simulink model "parallel_modules_2_parasitic"  (R2018a)
settings: Solver=FixedStepDiscrete  StartTime=0.0  StopTime=Tfinal  FixedStep=SampleTime  RelTol=1e-3
values from neighbouring files (symbols this model uses):
  C1A = 5e-6    (= 5e-06)    [param_parallel_modules_2_parasitic.m]
  C1B = 5e-6    (= 5e-06)    [param_parallel_modules_2_parasitic.m]
  C1C = 5e-6    (= 5e-06)    [param_parallel_modules_2_parasitic.m]
  connector_ind = 0.6e-6    (= 6e-07)    [param_parallel_modules_2_parasitic.m]
  connector_ind1 = 0.6e-6    (= 6e-07)    [param_parallel_modules_2_parasitic.m]
  connector_ind2 = 1.2e-6    (= 1.2e-06)    [param_parallel_modules_2_parasitic.m]
  connector_res = 1e-3    (= 0.001)    [param_parallel_modules_2_parasitic.m]
  connector_res1 = 1e-3    (= 0.001)    [param_parallel_modules_2_parasitic.m]
  connector_res2 = 1e-3    (= 0.001)    [param_parallel_modules_2_parasitic.m]
  ESLA = 19e-9    (= 1.9e-08)    [param_parallel_modules_2_parasitic.m]
  ESLB = 19e-9    (= 1.9e-08)    [param_parallel_modules_2_parasitic.m]
  ESLC = 19e-9    (= 1.9e-08)    [param_parallel_modules_2_parasitic.m]
  ESRA = 21.1e-3    (= 0.0211)    [param_parallel_modules_2_parasitic.m]
  ESRB = 21.1e-3    (= 0.0211)    [param_parallel_modules_2_parasitic.m]
  ESRC = 21.1e-3    (= 0.0211)    [param_parallel_modules_2_parasitic.m]
  ffund = 50    [param_parallel_modules_2_parasitic.m]
  LABBot = 10.20e-9    (= 1.02e-08)    [param_parallel_modules_2_parasitic.m]
  LABot = 20.25e-9    (= 2.025e-08)    [param_parallel_modules_2_parasitic.m]
  LABTop = 18.30e-9    (= 1.83e-08)    [param_parallel_modules_2_parasitic.m]
  LAMid = 01.30e-9    (= 1.3e-09)    [param_parallel_modules_2_parasitic.m]
  LATop = 03.40e-9    (= 3.4e-09)    [param_parallel_modules_2_parasitic.m]
  LBBot = 20.38e-9    (= 2.038e-08)    [param_parallel_modules_2_parasitic.m]
  LBCBot = 11.14e-9    (= 1.114e-08)    [param_parallel_modules_2_parasitic.m]
  LBCTop = 21.84e-9    (= 2.184e-08)    [param_parallel_modules_2_parasitic.m]
  LBMid = 01.30e-9    (= 1.3e-09)    [param_parallel_modules_2_parasitic.m]
  LBTop = 03.38e-9    (= 3.38e-09)    [param_parallel_modules_2_parasitic.m]
  LCBot = 20.94e-9    (= 2.094e-08)    [param_parallel_modules_2_parasitic.m]
  LCMid = 01.30e-9    (= 1.3e-09)    [param_parallel_modules_2_parasitic.m]
  LCTop = 03.41e-9    (= 3.41e-09)    [param_parallel_modules_2_parasitic.m]
  Lin = 1e-6    (= 1e-06)    [param_parallel_modules_2_parasitic.m]
  Lload1 = Xload1/(2*pi*ffund)    [param_parallel_modules_2_parasitic.m]
  Lload2 = Xload2/(2*pi*ffund)    [param_parallel_modules_2_parasitic.m]
  ModulationIndex1 = 0.9    [param_parallel_modules_2_parasitic.m]
  ModulationIndex2 = 0.9    [param_parallel_modules_2_parasitic.m]
  Module1Phase = 0    [param_parallel_modules_2_parasitic.m]
  Module2Phase = 0    [param_parallel_modules_2_parasitic.m]
  RABBot = 1422e-6-662e-6    (= 0.00076)    [param_parallel_modules_2_parasitic.m]
  RABot = 6645e-6    (= 0.006645)    [param_parallel_modules_2_parasitic.m]
  RABTop = 1037e-6-611e-6    (= 0.000426)    [param_parallel_modules_2_parasitic.m]
  RAMid = 218.8e-6*2    (= 0.0004376)    [param_parallel_modules_2_parasitic.m]
  RATop = 854e-6    (= 0.000854)    [param_parallel_modules_2_parasitic.m]
  RBBot = 664e-6    (= 0.000664)    [param_parallel_modules_2_parasitic.m]
  RBCBot = 662e-6-595e-6    (= 6.7e-05)    [param_parallel_modules_2_parasitic.m]
  RBCTop = 867e-6-611e-6    (= 0.000256)    [param_parallel_modules_2_parasitic.m]
  RBMid = 218e-6*2    (= 0.000436)    [param_parallel_modules_2_parasitic.m]
  RBTop = 813e-6    (= 0.000813)    [param_parallel_modules_2_parasitic.m]
  RCBot = 664e-6    (= 0.000664)    [param_parallel_modules_2_parasitic.m]
  RCMid = 218.3e-6*2    (= 0.0004366)    [param_parallel_modules_2_parasitic.m]
  RCTop = 854e-6    (= 0.000854)    [param_parallel_modules_2_parasitic.m]
  Rin = 0.1    [param_parallel_modules_2_parasitic.m]
  Rload1 = Z1*PF1    [param_parallel_modules_2_parasitic.m]
  Rload2 = Z2*PF2    [param_parallel_modules_2_parasitic.m]
  SampleTime = 1e-8    (= 1e-08)    [param_parallel_modules_2_parasitic.m]
  Vin = Vdc + Idc*Rin+((Idc1*connector_res1+Idc2*connector_res2)/2)    (= 271.488888889)    [param_parallel_modules_2_parasitic.m]
libraries: powerlib x90, simulink x12, powerlib_meascontrol x2
settings Model: Creator=enes_  LastModifiedBy=enes_

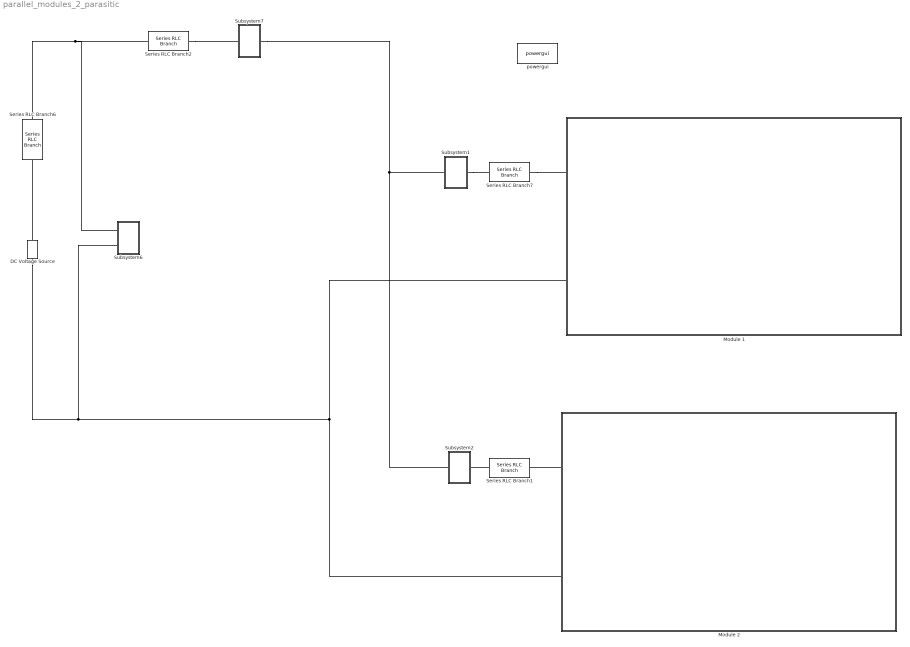
== system parallel_modules_2_parasitic ==
  DC Voltage Source : powerlib/Electrical Sources/DC Voltage Source  Amplitude=Vin  Measurements=None
  Module 1 : Subsystem
  Module 2 : Subsystem
  Series RLC Branch1 : powerlib/Elements/Series RLC Branch  LConnTagsString=__new0  RConnTagsString=__new0  BranchType=RL  Resistance=connector_res2  Inductance=connector_ind2  SetiL0=off  InitialCurrent=0  Capacitance=1e-6  Setx0=off  InitialVoltage=0  Measurements=None
  Series RLC Branch2 : powerlib/Elements/Series RLC Branch  LConnTagsString=__new0  RConnTagsString=__new0  BranchType=RL  Resistance=connector_res  Inductance=connector_ind  SetiL0=off  InitialCurrent=0  Capacitance=1e-6  Setx0=off  InitialVoltage=0  Measurements=None
  Series RLC Branch6 : powerlib/Elements/Series RLC Branch  LConnTagsString=__new0  RConnTagsString=__new0  BranchType=RL  Resistance=Rin  Inductance=Lin  SetiL0=off  InitialCurrent=0  Capacitance=C1A  Setx0=off  InitialVoltage=0  Measurements=None
  Series RLC Branch7 : powerlib/Elements/Series RLC Branch  LConnTagsString=__new0  RConnTagsString=__new0  BranchType=RL  Resistance=connector_res1  Inductance=connector_ind1  SetiL0=off  InitialCurrent=0  Capacitance=1e-6  Setx0=off  InitialVoltage=0  Measurements=None
  Subsystem1 : Subsystem
  Subsystem2 : Subsystem
  Subsystem6 : Subsystem
  Subsystem7 : Subsystem
  powergui : powerlib/powergui  Priority=1  SimulationMode=Discrete  SampleTime=SampleTime  frequency=60  Iterations=50  frequencyindice=0  Pbase=100e6  ErrMax=1e-4  UnitsV=kV  UnitsW=MW  buscounter=0  FunctionMessages=off  echomessages=off  EnableUseOfTLC=off  CurrentSourceSwitches=off  DisableSnubberDevices=off  DisableRonSwitches=off  DisableVfSwitches=off  DisplayEquations=off  SolverType=Tustin/Backward Euler (TBE)  Interpol=off  ExternalGateDelay=off  methode=off  Ts=100  x0status=blocks  SPID=off  SwTol=0  HookPort=off  RestoreLinks=warning  ResistiveCurrentMeasurement=off  Frange=[0:2:500]  Ylog=off  Xlog=on  ShowGrid=off  save=off  variable=ZData  structure=0  ZoomFFT=off  StartTime=0.0  cycles=1  DisplayStyle=1  fundamental=60  FreqAxis=off  MaxFrequency=1000  frequencyindicesteady=1  RmsSteady=1  display=off
  connections:
  DC Voltage Source/RConn1 -- Series RLC Branch6/RConn1
  Subsystem6/LConn1 -- Series RLC Branch2/LConn1 -- Series RLC Branch6/LConn1
  Subsystem6/LConn2 -- DC Voltage Source/LConn1 -- Module 1/LConn2 -- Module 2/LConn2
  Subsystem7/LConn1 -- Subsystem2/RConn1 -- Subsystem1/RConn1
  Series RLC Branch7/RConn1 -- Module 1/LConn1
  Module 2/LConn1 -- Series RLC Branch1/RConn1
  Series RLC Branch2/RConn1 -- Subsystem7/RConn1
  Subsystem1/LConn1 -- Series RLC Branch7/LConn1
  Series RLC Branch1/LConn1 -- Subsystem2/LConn1

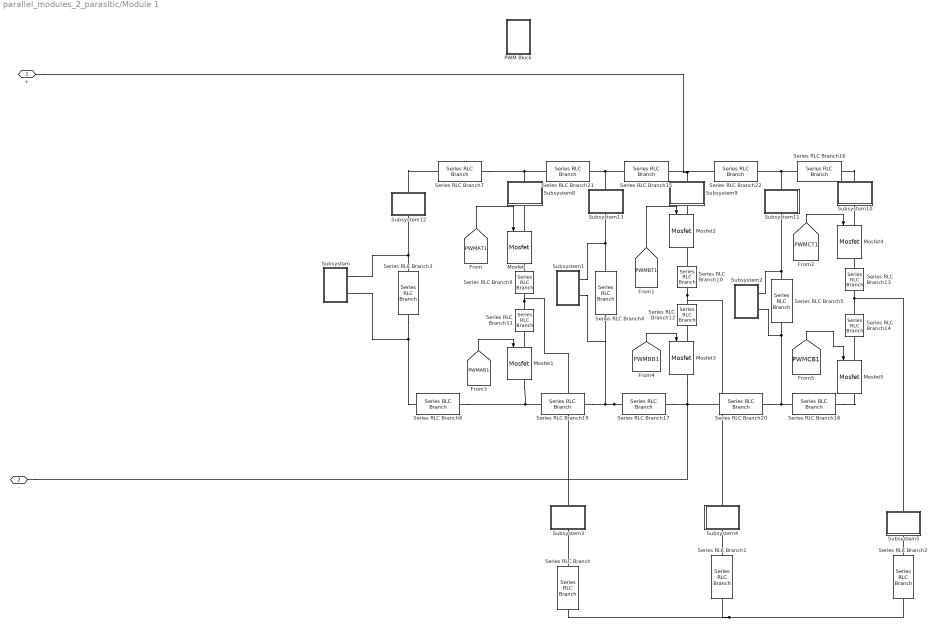
== system parallel_modules_2_parasitic/Module 1 ==
  Mosfet{,1..5} (6 alike) : powerlib/Power Electronics/Mosfet  Ron=0.1  Lon=0  Rd=0.01  Vfd=0  IC=0  Rs=1e5  Cs=inf  Measurements=on
  PWM Block : Subsystem
  Series RLC Branch : powerlib/Elements/Series RLC Branch  LConnTagsString=__new0  RConnTagsString=__new0  BranchType=RL  Resistance=Rload1  Inductance=Lload1  SetiL0=off  InitialCurrent=0  Capacitance=1e-6  Setx0=off  InitialVoltage=0  Measurements=None
  Series RLC Branch1 : powerlib/Elements/Series RLC Branch  LConnTagsString=__new0  RConnTagsString=__new0  BranchType=RL  Resistance=Rload1  Inductance=Lload1  SetiL0=off  InitialCurrent=0  Capacitance=1e-6  Setx0=off  InitialVoltage=0  Measurements=None
  Series RLC Branch10 : powerlib/Elements/Series RLC Branch  LConnTagsString=__new0  RConnTagsString=__new0  BranchType=RL  Resistance=RBMid/2  Inductance=LBMid/2  SetiL0=off  InitialCurrent=0  Capacitance=1e-6  Setx0=off  InitialVoltage=0  Measurements=None
  Series RLC Branch11 : powerlib/Elements/Series RLC Branch  LConnTagsString=__new0  RConnTagsString=__new0  BranchType=RL  Resistance=RAMid/2  Inductance=LAMid/2  SetiL0=off  InitialCurrent=0  Capacitance=1e-6  Setx0=off  InitialVoltage=0  Measurements=None
  Series RLC Branch12 : powerlib/Elements/Series RLC Branch  LConnTagsString=__new0  RConnTagsString=__new0  BranchType=RL  Resistance=RBMid/2  Inductance=LBMid/2  SetiL0=off  InitialCurrent=0  Capacitance=1e-6  Setx0=off  InitialVoltage=0  Measurements=None
  Series RLC Branch13 : powerlib/Elements/Series RLC Branch  LConnTagsString=__new0  RConnTagsString=__new0  BranchType=RL  Resistance=RCMid/2  Inductance=LCMid/2  SetiL0=off  InitialCurrent=0  Capacitance=1e-6  Setx0=off  InitialVoltage=0  Measurements=None
  Series RLC Branch14 : powerlib/Elements/Series RLC Branch  LConnTagsString=__new0  RConnTagsString=__new0  BranchType=RL  Resistance=RCMid/2  Inductance=LCMid/2  SetiL0=off  InitialCurrent=0  Capacitance=1e-6  Setx0=off  InitialVoltage=0  Measurements=None
  Series RLC Branch15 : powerlib/Elements/Series RLC Branch  LConnTagsString=__new0  RConnTagsString=__new0  BranchType=RL  Resistance=RBTop  Inductance=LBTop  SetiL0=off  InitialCurrent=0  Capacitance=1e-6  Setx0=off  InitialVoltage=0  Measurements=None
  Series RLC Branch16 : powerlib/Elements/Series RLC Branch  LConnTagsString=__new0  RConnTagsString=__new0  BranchType=RL  Resistance=RCTop  Inductance=LCTop  SetiL0=off  InitialCurrent=0  Capacitance=1e-6  Setx0=off  InitialVoltage=0  Measurements=None
  Series RLC Branch17 : powerlib/Elements/Series RLC Branch  LConnTagsString=__new0  RConnTagsString=__new0  BranchType=RL  Resistance=RBBot  Inductance=LBBot  SetiL0=off  InitialCurrent=0  Capacitance=1e-6  Setx0=off  InitialVoltage=0  Measurements=None
  Series RLC Branch18 : powerlib/Elements/Series RLC Branch  LConnTagsString=__new0  RConnTagsString=__new0  BranchType=RL  Resistance=RCBot  Inductance=LCBot  SetiL0=off  InitialCurrent=0  Capacitance=1e-6  Setx0=off  InitialVoltage=0  Measurements=None
  Series RLC Branch19 : powerlib/Elements/Series RLC Branch  LConnTagsString=__new0  RConnTagsString=__new0  BranchType=RL  Resistance=RABBot  Inductance=LABBot  SetiL0=off  InitialCurrent=0  Capacitance=1e-6  Setx0=off  InitialVoltage=0  Measurements=None
  Series RLC Branch2 : powerlib/Elements/Series RLC Branch  LConnTagsString=__new0  RConnTagsString=__new0  BranchType=RL  Resistance=Rload1  Inductance=Lload1  SetiL0=off  InitialCurrent=0  Capacitance=1e-6  Setx0=off  InitialVoltage=0  Measurements=None
  Series RLC Branch20 : powerlib/Elements/Series RLC Branch  LConnTagsString=__new0  RConnTagsString=__new0  BranchType=RL  Resistance=RBCBot  Inductance=LBCBot  SetiL0=off  InitialCurrent=0  Capacitance=1e-6  Setx0=off  InitialVoltage=0  Measurements=None
  Series RLC Branch21 : powerlib/Elements/Series RLC Branch  LConnTagsString=__new0  RConnTagsString=__new0  BranchType=RL  Resistance=RABTop  Inductance=LABTop  SetiL0=off  InitialCurrent=0  Capacitance=1e-6  Setx0=off  InitialVoltage=0  Measurements=None
  Series RLC Branch22 : powerlib/Elements/Series RLC Branch  LConnTagsString=__new0  RConnTagsString=__new0  BranchType=RL  Resistance=RBCTop  Inductance=LBCTop  SetiL0=off  InitialCurrent=0  Capacitance=1e-6  Setx0=off  InitialVoltage=0  Measurements=None
  Series RLC Branch3 : powerlib/Elements/Series RLC Branch  LConnTagsString=__new0  RConnTagsString=__new0  BranchType=RLC  Resistance=ESRA  Inductance=ESLA  SetiL0=off  InitialCurrent=0  Capacitance=C1A  Setx0=off  InitialVoltage=0  Measurements=None
  Series RLC Branch4 : powerlib/Elements/Series RLC Branch  LConnTagsString=__new0  RConnTagsString=__new0  BranchType=RLC  Resistance=ESRB  Inductance=ESLB  SetiL0=off  InitialCurrent=0  Capacitance=C1B  Setx0=off  InitialVoltage=0  Measurements=None
  Series RLC Branch5 : powerlib/Elements/Series RLC Branch  LConnTagsString=__new0  RConnTagsString=__new0  BranchType=RLC  Resistance=ESRC  Inductance=ESLC  SetiL0=off  InitialCurrent=0  Capacitance=C1C  Setx0=off  InitialVoltage=0  Measurements=None
  Series RLC Branch7 : powerlib/Elements/Series RLC Branch  LConnTagsString=__new0  RConnTagsString=__new0  BranchType=RL  Resistance=RATop  Inductance=LATop  SetiL0=off  InitialCurrent=0  Capacitance=1e-6  Setx0=off  InitialVoltage=0  Measurements=None
  Series RLC Branch8 : powerlib/Elements/Series RLC Branch  LConnTagsString=__new0  RConnTagsString=__new0  BranchType=RL  Resistance=RABot  Inductance=LABot  SetiL0=off  InitialCurrent=0  Capacitance=1e-6  Setx0=off  InitialVoltage=0  Measurements=None
  Series RLC Branch9 : powerlib/Elements/Series RLC Branch  LConnTagsString=__new0  RConnTagsString=__new0  BranchType=RL  Resistance=RAMid/2  Inductance=LAMid/2  SetiL0=off  InitialCurrent=0  Capacitance=1e-6  Setx0=off  InitialVoltage=0  Measurements=None
  Subsystem : Subsystem
  Subsystem1 : Subsystem
  Subsystem10 : Subsystem
  Subsystem11 : Subsystem
  Subsystem12 : Subsystem
  Subsystem13 : Subsystem
  Subsystem2 : Subsystem
  Subsystem3 : Subsystem
  Subsystem4 : Subsystem
  Subsystem5 : Subsystem
  Subsystem8 : Subsystem
  Subsystem9 : Subsystem
  + : PMIOPort  Side=Left
  - : PMIOPort  Port=2  Side=Left
  wires:
  [PWMAT1] -> Mosfet/1
  [PWMAB1] -> Mosfet1/1
  [PWMBT1] -> Mosfet2/1
  [PWMCB1] -> Mosfet5/1
  [PWMBB1] -> Mosfet3/1
  [PWMCT1] -> Mosfet4/1
  connections:
  Series RLC Branch13/LConn1 -- Mosfet4/RConn1
  Subsystem/LConn2 -- Series RLC Branch8/LConn1 -- Series RLC Branch3/RConn1
  Series RLC Branch21/LConn1 -- Subsystem8/RConn1 -- Series RLC Branch7/RConn1
  Series RLC Branch16/LConn1 -- Subsystem11/RConn1 -- Series RLC Branch22/RConn1
  Series RLC Branch11/LConn1 -- Subsystem3/RConn1 -- Series RLC Branch9/RConn1
  Mosfet4/LConn1 -- Subsystem10/LConn1
  Series RLC Branch8/RConn1 -- Mosfet1/RConn1 -- Series RLC Branch19/LConn1
  Subsystem2/LConn1 -- Series RLC Branch5/LConn1 -- Subsystem11/LConn1
  Series RLC Branch17/RConn1 -- -/RConn1 -- Mosfet3/RConn1 -- Series RLC Branch20/LConn1
  Series RLC Branch12/LConn1 -- Subsystem4/RConn1 -- Series RLC Branch10/RConn1
  Series RLC Branch15/LConn1 -- Subsystem13/RConn1 -- Series RLC Branch21/RConn1
  Series RLC Branch18/RConn1 -- Mosfet5/RConn1
  Mosfet3/LConn1 -- Series RLC Branch12/RConn1
  Series RLC Branch/RConn1 -- Series RLC Branch2/RConn1 -- Series RLC Branch1/RConn1
  Subsystem/LConn1 -- Subsystem12/LConn1 -- Series RLC Branch3/LConn1
  Series RLC Branch13/RConn1 -- Series RLC Branch14/LConn1 -- Subsystem5/RConn1
  Subsystem9/LConn1 -- Mosfet2/LConn1
  Subsystem10/RConn1 -- Series RLC Branch16/RConn1
  Series RLC Branch9/LConn1 -- Mosfet/RConn1
  Series RLC Branch17/LConn1 -- Subsystem1/LConn2 -- Series RLC Branch4/RConn1 -- Series RLC Branch19/RConn1
  Series RLC Branch1/LConn1 -- Subsystem4/LConn1
  Mosfet/LConn1 -- Subsystem8/LConn1
  Mosfet1/LConn1 -- Series RLC Branch11/RConn1
  Series RLC Branch2/LConn1 -- Subsystem5/LConn1
  Subsystem12/RConn1 -- Series RLC Branch7/LConn1
  Subsystem1/LConn1 -- Subsystem13/LConn1 -- Series RLC Branch4/LConn1
  Series RLC Branch10/LConn1 -- Mosfet2/RConn1
  +/RConn1 -- Series RLC Branch15/RConn1 -- Series RLC Branch22/LConn1 -- Subsystem9/RConn1
  Mosfet5/LConn1 -- Series RLC Branch14/RConn1
  Series RLC Branch5/RConn1 -- Subsystem2/LConn2 -- Series RLC Branch20/RConn1 -- Series RLC Branch18/LConn1
  Series RLC Branch/LConn1 -- Subsystem3/LConn1

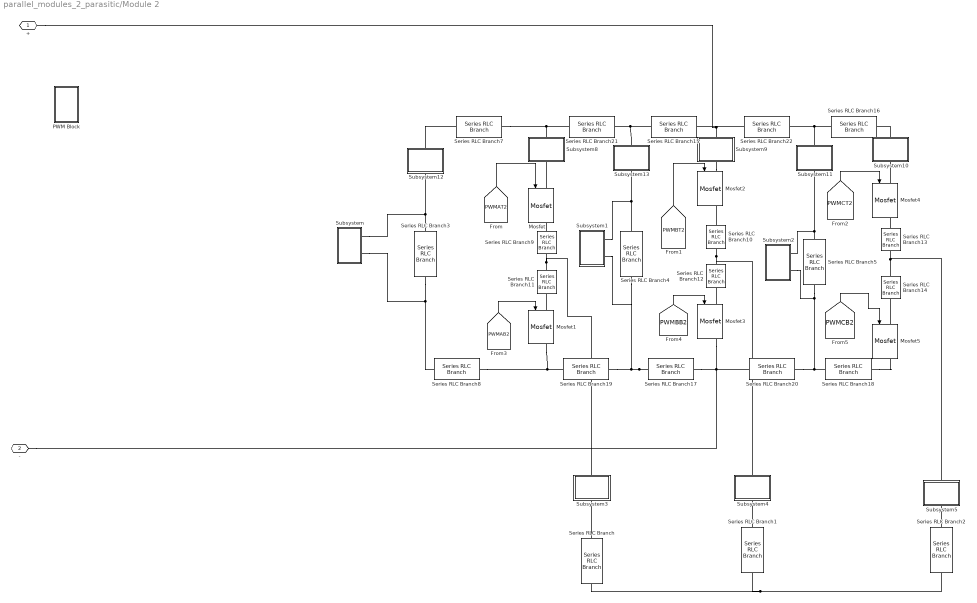
== system parallel_modules_2_parasitic/Module 2 ==
  Mosfet{,1..5} (6 alike) : powerlib/Power Electronics/Mosfet  Ron=0.1  Lon=0  Rd=0.01  Vfd=0  IC=0  Rs=1e5  Cs=inf  Measurements=on
  PWM Block : Subsystem
  Series RLC Branch : powerlib/Elements/Series RLC Branch  LConnTagsString=__new0  RConnTagsString=__new0  BranchType=RL  Resistance=Rload2  Inductance=Lload2  SetiL0=off  InitialCurrent=0  Capacitance=1e-6  Setx0=off  InitialVoltage=0  Measurements=None
  Series RLC Branch1 : powerlib/Elements/Series RLC Branch  LConnTagsString=__new0  RConnTagsString=__new0  BranchType=RL  Resistance=Rload2  Inductance=Lload2  SetiL0=off  InitialCurrent=0  Capacitance=1e-6  Setx0=off  InitialVoltage=0  Measurements=None
  Series RLC Branch10 : powerlib/Elements/Series RLC Branch  LConnTagsString=__new0  RConnTagsString=__new0  BranchType=RL  Resistance=RBMid/2  Inductance=LBMid/2  SetiL0=off  InitialCurrent=0  Capacitance=1e-6  Setx0=off  InitialVoltage=0  Measurements=None
  Series RLC Branch11 : powerlib/Elements/Series RLC Branch  LConnTagsString=__new0  RConnTagsString=__new0  BranchType=RL  Resistance=RAMid/2  Inductance=LAMid/2  SetiL0=off  InitialCurrent=0  Capacitance=1e-6  Setx0=off  InitialVoltage=0  Measurements=None
  Series RLC Branch12 : powerlib/Elements/Series RLC Branch  LConnTagsString=__new0  RConnTagsString=__new0  BranchType=RL  Resistance=RBMid/2  Inductance=LBMid/2  SetiL0=off  InitialCurrent=0  Capacitance=1e-6  Setx0=off  InitialVoltage=0  Measurements=None
  Series RLC Branch13 : powerlib/Elements/Series RLC Branch  LConnTagsString=__new0  RConnTagsString=__new0  BranchType=RL  Resistance=RCMid/2  Inductance=LCMid/2  SetiL0=off  InitialCurrent=0  Capacitance=1e-6  Setx0=off  InitialVoltage=0  Measurements=None
  Series RLC Branch14 : powerlib/Elements/Series RLC Branch  LConnTagsString=__new0  RConnTagsString=__new0  BranchType=RL  Resistance=RCMid/2  Inductance=LCMid/2  SetiL0=off  InitialCurrent=0  Capacitance=1e-6  Setx0=off  InitialVoltage=0  Measurements=None
  Series RLC Branch15 : powerlib/Elements/Series RLC Branch  LConnTagsString=__new0  RConnTagsString=__new0  BranchType=RL  Resistance=RBTop  Inductance=LBTop  SetiL0=off  InitialCurrent=0  Capacitance=1e-6  Setx0=off  InitialVoltage=0  Measurements=None
  Series RLC Branch16 : powerlib/Elements/Series RLC Branch  LConnTagsString=__new0  RConnTagsString=__new0  BranchType=RL  Resistance=RCTop  Inductance=LCTop  SetiL0=off  InitialCurrent=0  Capacitance=1e-6  Setx0=off  InitialVoltage=0  Measurements=None
  Series RLC Branch17 : powerlib/Elements/Series RLC Branch  LConnTagsString=__new0  RConnTagsString=__new0  BranchType=RL  Resistance=RBBot  Inductance=LBBot  SetiL0=off  InitialCurrent=0  Capacitance=1e-6  Setx0=off  InitialVoltage=0  Measurements=None
  Series RLC Branch18 : powerlib/Elements/Series RLC Branch  LConnTagsString=__new0  RConnTagsString=__new0  BranchType=RL  Resistance=RCBot  Inductance=LCBot  SetiL0=off  InitialCurrent=0  Capacitance=1e-6  Setx0=off  InitialVoltage=0  Measurements=None
  Series RLC Branch19 : powerlib/Elements/Series RLC Branch  LConnTagsString=__new0  RConnTagsString=__new0  BranchType=RL  Resistance=RABBot  Inductance=LABBot  SetiL0=off  InitialCurrent=0  Capacitance=1e-6  Setx0=off  InitialVoltage=0  Measurements=None
  Series RLC Branch2 : powerlib/Elements/Series RLC Branch  LConnTagsString=__new0  RConnTagsString=__new0  BranchType=RL  Resistance=Rload2  Inductance=Lload2  SetiL0=off  InitialCurrent=0  Capacitance=1e-6  Setx0=off  InitialVoltage=0  Measurements=None
  Series RLC Branch20 : powerlib/Elements/Series RLC Branch  LConnTagsString=__new0  RConnTagsString=__new0  BranchType=RL  Resistance=RBCBot  Inductance=LBCBot  SetiL0=off  InitialCurrent=0  Capacitance=1e-6  Setx0=off  InitialVoltage=0  Measurements=None
  Series RLC Branch21 : powerlib/Elements/Series RLC Branch  LConnTagsString=__new0  RConnTagsString=__new0  BranchType=RL  Resistance=RABTop  Inductance=LABTop  SetiL0=off  InitialCurrent=0  Capacitance=1e-6  Setx0=off  InitialVoltage=0  Measurements=None
  Series RLC Branch22 : powerlib/Elements/Series RLC Branch  LConnTagsString=__new0  RConnTagsString=__new0  BranchType=RL  Resistance=RBCTop  Inductance=LBCTop  SetiL0=off  InitialCurrent=0  Capacitance=1e-6  Setx0=off  InitialVoltage=0  Measurements=None
  Series RLC Branch3 : powerlib/Elements/Series RLC Branch  LConnTagsString=__new0  RConnTagsString=__new0  BranchType=RLC  Resistance=ESRA  Inductance=ESLA  SetiL0=off  InitialCurrent=0  Capacitance=C1A  Setx0=off  InitialVoltage=0  Measurements=None
  Series RLC Branch4 : powerlib/Elements/Series RLC Branch  LConnTagsString=__new0  RConnTagsString=__new0  BranchType=RLC  Resistance=ESRB  Inductance=ESLB  SetiL0=off  InitialCurrent=0  Capacitance=C1B  Setx0=off  InitialVoltage=0  Measurements=None
  Series RLC Branch5 : powerlib/Elements/Series RLC Branch  LConnTagsString=__new0  RConnTagsString=__new0  BranchType=RLC  Resistance=ESRC  Inductance=ESLC  SetiL0=off  InitialCurrent=0  Capacitance=C1C  Setx0=off  InitialVoltage=0  Measurements=None
  Series RLC Branch7 : powerlib/Elements/Series RLC Branch  LConnTagsString=__new0  RConnTagsString=__new0  BranchType=RL  Resistance=RATop  Inductance=LATop  SetiL0=off  InitialCurrent=0  Capacitance=1e-6  Setx0=off  InitialVoltage=0  Measurements=None
  Series RLC Branch8 : powerlib/Elements/Series RLC Branch  LConnTagsString=__new0  RConnTagsString=__new0  BranchType=RL  Resistance=RABot  Inductance=LABot  SetiL0=off  InitialCurrent=0  Capacitance=1e-6  Setx0=off  InitialVoltage=0  Measurements=None
  Series RLC Branch9 : powerlib/Elements/Series RLC Branch  LConnTagsString=__new0  RConnTagsString=__new0  BranchType=RL  Resistance=RAMid/2  Inductance=LAMid/2  SetiL0=off  InitialCurrent=0  Capacitance=1e-6  Setx0=off  InitialVoltage=0  Measurements=None
  Subsystem : Subsystem
  Subsystem1 : Subsystem
  Subsystem10 : Subsystem
  Subsystem11 : Subsystem
  Subsystem12 : Subsystem
  Subsystem13 : Subsystem
  Subsystem2 : Subsystem
  Subsystem3 : Subsystem
  Subsystem4 : Subsystem
  Subsystem5 : Subsystem
  Subsystem8 : Subsystem
  Subsystem9 : Subsystem
  + : PMIOPort  Side=Left
  - : PMIOPort  Port=2  Side=Left
  wires:
  [PWMAT2] -> Mosfet/1
  [PWMAB2] -> Mosfet1/1
  [PWMBT2] -> Mosfet2/1
  [PWMCB2] -> Mosfet5/1
  [PWMBB2] -> Mosfet3/1
  [PWMCT2] -> Mosfet4/1
  connections:
  Series RLC Branch13/LConn1 -- Mosfet4/RConn1
  Subsystem/LConn2 -- Series RLC Branch8/LConn1 -- Series RLC Branch3/RConn1
  Series RLC Branch21/LConn1 -- Subsystem8/RConn1 -- Series RLC Branch7/RConn1
  Series RLC Branch16/LConn1 -- Subsystem11/RConn1 -- Series RLC Branch22/RConn1
  Series RLC Branch11/LConn1 -- Subsystem3/RConn1 -- Series RLC Branch9/RConn1
  Mosfet4/LConn1 -- Subsystem10/LConn1
  Series RLC Branch8/RConn1 -- Mosfet1/RConn1 -- Series RLC Branch19/LConn1
  Subsystem2/LConn1 -- Series RLC Branch5/LConn1 -- Subsystem11/LConn1
  Series RLC Branch17/RConn1 -- Mosfet3/RConn1 -- Series RLC Branch20/LConn1 -- -/RConn1
  Series RLC Branch12/LConn1 -- Subsystem4/RConn1 -- Series RLC Branch10/RConn1
  Series RLC Branch15/LConn1 -- Subsystem13/RConn1 -- Series RLC Branch21/RConn1
  Series RLC Branch18/RConn1 -- Mosfet5/RConn1
  Mosfet3/LConn1 -- Series RLC Branch12/RConn1
  Series RLC Branch/RConn1 -- Series RLC Branch2/RConn1 -- Series RLC Branch1/RConn1
  Subsystem/LConn1 -- Subsystem12/LConn1 -- Series RLC Branch3/LConn1
  Series RLC Branch13/RConn1 -- Series RLC Branch14/LConn1 -- Subsystem5/RConn1
  Subsystem9/LConn1 -- Mosfet2/LConn1
  Subsystem10/RConn1 -- Series RLC Branch16/RConn1
  Series RLC Branch9/LConn1 -- Mosfet/RConn1
  Series RLC Branch17/LConn1 -- Subsystem1/LConn2 -- Series RLC Branch4/RConn1 -- Series RLC Branch19/RConn1
  Series RLC Branch1/LConn1 -- Subsystem4/LConn1
  Mosfet/LConn1 -- Subsystem8/LConn1
  Mosfet1/LConn1 -- Series RLC Branch11/RConn1
  Series RLC Branch2/LConn1 -- Subsystem5/LConn1
  Subsystem12/RConn1 -- Series RLC Branch7/LConn1
  Subsystem1/LConn1 -- Subsystem13/LConn1 -- Series RLC Branch4/LConn1
  Series RLC Branch10/LConn1 -- Mosfet2/RConn1
  Series RLC Branch22/LConn1 -- Subsystem9/RConn1 -- Series RLC Branch15/RConn1 -- +/RConn1
  Mosfet5/LConn1 -- Series RLC Branch14/RConn1
  Series RLC Branch5/RConn1 -- Subsystem2/LConn2 -- Series RLC Branch20/RConn1 -- Series RLC Branch18/LConn1
  Series RLC Branch/LConn1 -- Subsystem3/LConn1

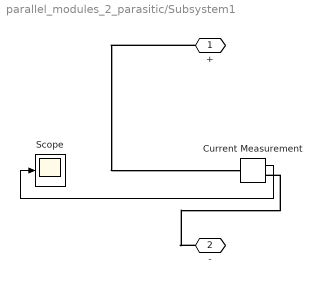
== system parallel_modules_2_parasitic/Subsystem1 ==
  Current Measurement : powerlib/Measurements/Current Measurement  PhasorSimulation=off  OutputType=Complex  PSBequivalent=0
  Scope : Scope
  + : PMIOPort  Side=Right
  - : PMIOPort  Port=2  Side=Left
  wires:
  Current Measurement/1 -> Scope/1
  connections:
  +/RConn1 -- Current Measurement/LConn1
  -/RConn1 -- Current Measurement/RConn1

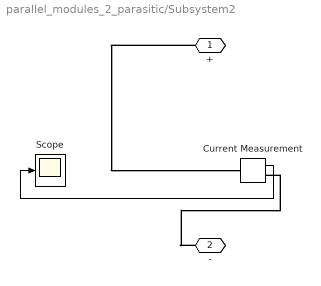
== system parallel_modules_2_parasitic/Subsystem2 ==
  Current Measurement : powerlib/Measurements/Current Measurement  PhasorSimulation=off  OutputType=Complex  PSBequivalent=0
  Scope : Scope
  + : PMIOPort  Side=Right
  - : PMIOPort  Port=2  Side=Left
  wires:
  Current Measurement/1 -> Scope/1
  connections:
  +/RConn1 -- Current Measurement/LConn1
  -/RConn1 -- Current Measurement/RConn1

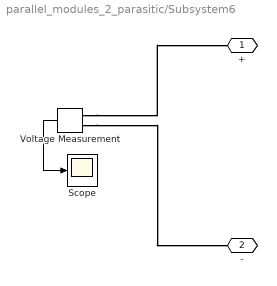
== system parallel_modules_2_parasitic/Subsystem6 ==
  Scope : Scope
  Voltage Measurement : powerlib/Measurements/Voltage Measurement  PhasorSimulation=off  OutputType=Complex  PSBequivalent=0
  + : PMIOPort  Side=Left
  - : PMIOPort  Port=2  Side=Left
  wires:
  Voltage Measurement/1 -> Scope/1
  connections:
  Voltage Measurement/LConn1 -- +/RConn1
  Voltage Measurement/LConn2 -- -/RConn1

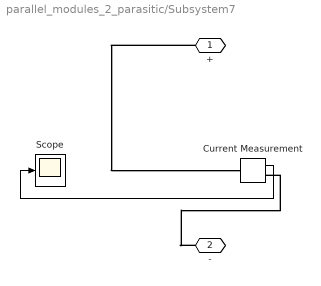
== system parallel_modules_2_parasitic/Subsystem7 ==
  Current Measurement : powerlib/Measurements/Current Measurement  PhasorSimulation=off  OutputType=Complex  PSBequivalent=0
  Scope : Scope
  + : PMIOPort  Side=Right
  - : PMIOPort  Port=2  Side=Left
  wires:
  Current Measurement/1 -> Scope/1
  connections:
  +/RConn1 -- Current Measurement/LConn1
  -/RConn1 -- Current Measurement/RConn1

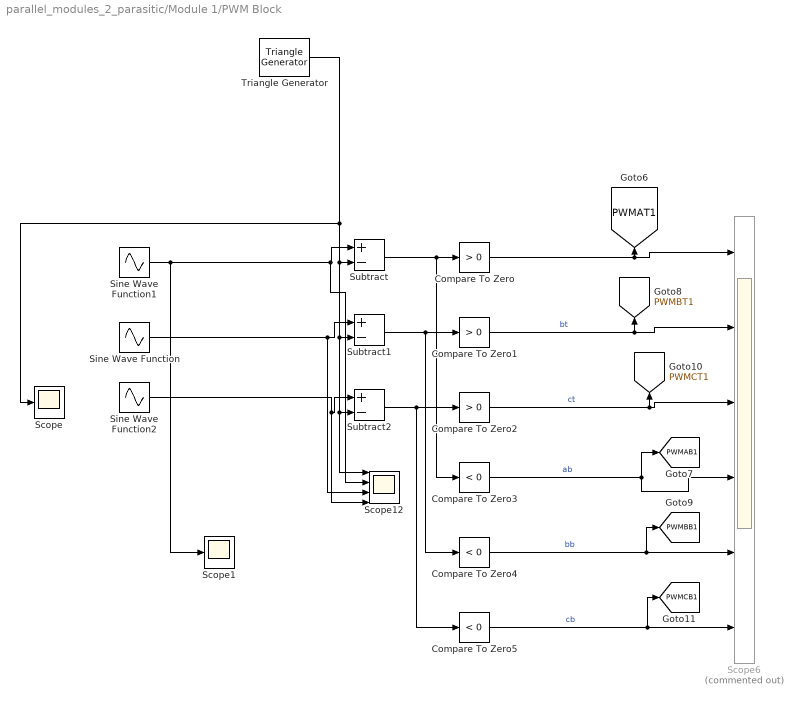
== system parallel_modules_2_parasitic/Module 1/PWM Block ==
  Compare To Zero : simulink/Logic and Bit Operations/Compare To Zero  relop=>  OutDataTypeStr=boolean
  Compare To Zero1 : simulink/Logic and Bit Operations/Compare To Zero  relop=>  OutDataTypeStr=boolean
  Compare To Zero2 : simulink/Logic and Bit Operations/Compare To Zero  relop=>  OutDataTypeStr=boolean
  Compare To Zero3 : simulink/Logic and Bit Operations/Compare To Zero  relop=<  OutDataTypeStr=boolean
  Compare To Zero4 : simulink/Logic and Bit Operations/Compare To Zero  relop=<  OutDataTypeStr=boolean
  Compare To Zero5 : simulink/Logic and Bit Operations/Compare To Zero  relop=<  OutDataTypeStr=boolean
  Scope : Scope
  Scope1 : Scope
  Scope12 : Scope  NumInputPorts=4
  Scope6 : Scope  Commented=on  NumInputPorts=6
  Sine Wave Function : Sin  Amplitude=ModulationIndex1  Frequency=ffund*2*pi  Phase=-2*pi/3  SampleTime=0
  Sine Wave Function1 : Sin  Amplitude=ModulationIndex1  Frequency=ffund*2*pi  SampleTime=0
  Sine Wave Function2 : Sin  Amplitude=ModulationIndex1  Frequency=ffund*2*pi  Phase=2*pi/3  SampleTime=0
  Subtract : Sum  Inputs=+-
  Subtract1 : Sum  Inputs=+-
  Subtract2 : Sum  Inputs=+-
  Triangle Generator : powerlib_meascontrol/Pulse & Signal Generators/Triangle Generator  Freq=fsw  Phase=Module1Phase  Ts=SampleTime
  tag scope: PWMAB1=global, PWMAT1=global, PWMBB1=global, PWMBT1=global, PWMCB1=global, PWMCT1=global
  wires:
  Compare To Zero2/1 -> [PWMCT1], Scope6/3  "ct"
  Sine Wave Function/1 -> Subtract1/1, Scope12/3
  Subtract2/1 -> Compare To Zero5/1, Compare To Zero2/1
  Sine Wave Function1/1 -> Scope1/1, Scope12/2, Subtract/1
  Subtract1/1 -> Compare To Zero4/1, Compare To Zero1/1
  Triangle Generator/1 -> Scope/1, Scope12/1, Subtract2/2, Subtract1/2, Subtract/2
  Compare To Zero/1 -> Scope6/1, [PWMAT1]
  Subtract/1 -> Compare To Zero3/1, Compare To Zero/1
  Compare To Zero1/1 -> [PWMBT1], Scope6/2  "bt"
  Compare To Zero5/1 -> [PWMCB1], Scope6/6  "cb"
  Compare To Zero4/1 -> [PWMBB1], Scope6/5  "bb"
  Sine Wave Function2/1 -> Scope12/4, Subtract2/1
  Compare To Zero3/1 -> [PWMAB1], Scope6/4  "ab"

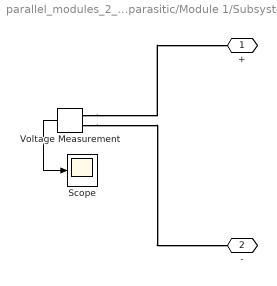
== system parallel_modules_2_parasitic/Module 1/Subsystem ==
  Scope : Scope
  Voltage Measurement : powerlib/Measurements/Voltage Measurement  PhasorSimulation=off  OutputType=Complex  PSBequivalent=0
  + : PMIOPort  Side=Left
  - : PMIOPort  Port=2  Side=Left
  wires:
  Voltage Measurement/1 -> Scope/1
  connections:
  Voltage Measurement/LConn1 -- +/RConn1
  Voltage Measurement/LConn2 -- -/RConn1

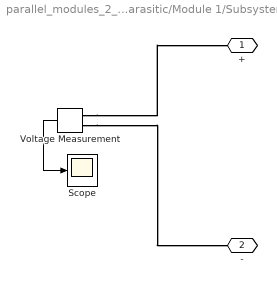
== system parallel_modules_2_parasitic/Module 1/Subsystem1 ==
  Scope : Scope
  Voltage Measurement : powerlib/Measurements/Voltage Measurement  PhasorSimulation=off  OutputType=Complex  PSBequivalent=0
  + : PMIOPort  Side=Left
  - : PMIOPort  Port=2  Side=Left
  wires:
  Voltage Measurement/1 -> Scope/1
  connections:
  Voltage Measurement/LConn1 -- +/RConn1
  Voltage Measurement/LConn2 -- -/RConn1

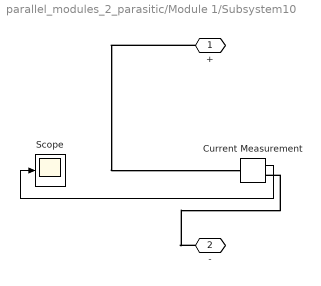
== system parallel_modules_2_parasitic/Module 1/Subsystem10 ==
  Current Measurement : powerlib/Measurements/Current Measurement  PhasorSimulation=off  OutputType=Complex  PSBequivalent=0
  Scope : Scope
  + : PMIOPort  Side=Right
  - : PMIOPort  Port=2  Side=Left
  wires:
  Current Measurement/1 -> Scope/1
  connections:
  +/RConn1 -- Current Measurement/LConn1
  -/RConn1 -- Current Measurement/RConn1

== system parallel_modules_2_parasitic/Module 1/Subsystem11 ==
  Current Measurement : powerlib/Measurements/Current Measurement  PhasorSimulation=off  OutputType=Complex  PSBequivalent=0
  Scope : Scope
  + : PMIOPort  Side=Right
  - : PMIOPort  Port=2  Side=Left
  wires:
  Current Measurement/1 -> Scope/1
  connections:
  +/RConn1 -- Current Measurement/LConn1
  -/RConn1 -- Current Measurement/RConn1

== system parallel_modules_2_parasitic/Module 1/Subsystem12 ==
  Current Measurement : powerlib/Measurements/Current Measurement  PhasorSimulation=off  OutputType=Complex  PSBequivalent=0
  Scope : Scope
  + : PMIOPort  Side=Right
  - : PMIOPort  Port=2  Side=Left
  wires:
  Current Measurement/1 -> Scope/1
  connections:
  +/RConn1 -- Current Measurement/LConn1
  -/RConn1 -- Current Measurement/RConn1

== system parallel_modules_2_parasitic/Module 1/Subsystem13 ==
  Current Measurement : powerlib/Measurements/Current Measurement  PhasorSimulation=off  OutputType=Complex  PSBequivalent=0
  Scope : Scope
  + : PMIOPort  Side=Right
  - : PMIOPort  Port=2  Side=Left
  wires:
  Current Measurement/1 -> Scope/1
  connections:
  +/RConn1 -- Current Measurement/LConn1
  -/RConn1 -- Current Measurement/RConn1

== system parallel_modules_2_parasitic/Module 1/Subsystem2 ==
  Scope : Scope
  Voltage Measurement : powerlib/Measurements/Voltage Measurement  PhasorSimulation=off  OutputType=Complex  PSBequivalent=0
  + : PMIOPort  Side=Left
  - : PMIOPort  Port=2  Side=Left
  wires:
  Voltage Measurement/1 -> Scope/1
  connections:
  Voltage Measurement/LConn1 -- +/RConn1
  Voltage Measurement/LConn2 -- -/RConn1

== system parallel_modules_2_parasitic/Module 1/Subsystem3 ==
  Current Measurement : powerlib/Measurements/Current Measurement  PhasorSimulation=off  OutputType=Complex  PSBequivalent=0
  Scope : Scope
  + : PMIOPort  Side=Right
  - : PMIOPort  Port=2  Side=Left
  wires:
  Current Measurement/1 -> Scope/1
  connections:
  +/RConn1 -- Current Measurement/LConn1
  -/RConn1 -- Current Measurement/RConn1

== system parallel_modules_2_parasitic/Module 1/Subsystem4 ==
  Current Measurement : powerlib/Measurements/Current Measurement  PhasorSimulation=off  OutputType=Complex  PSBequivalent=0
  Scope : Scope
  + : PMIOPort  Side=Right
  - : PMIOPort  Port=2  Side=Left
  wires:
  Current Measurement/1 -> Scope/1
  connections:
  +/RConn1 -- Current Measurement/LConn1
  -/RConn1 -- Current Measurement/RConn1

== system parallel_modules_2_parasitic/Module 1/Subsystem5 ==
  Current Measurement : powerlib/Measurements/Current Measurement  PhasorSimulation=off  OutputType=Complex  PSBequivalent=0
  Scope : Scope
  + : PMIOPort  Side=Right
  - : PMIOPort  Port=2  Side=Left
  wires:
  Current Measurement/1 -> Scope/1
  connections:
  +/RConn1 -- Current Measurement/LConn1
  -/RConn1 -- Current Measurement/RConn1

== system parallel_modules_2_parasitic/Module 1/Subsystem8 ==
  Current Measurement : powerlib/Measurements/Current Measurement  PhasorSimulation=off  OutputType=Complex  PSBequivalent=0
  Scope : Scope
  + : PMIOPort  Side=Right
  - : PMIOPort  Port=2  Side=Left
  wires:
  Current Measurement/1 -> Scope/1
  connections:
  +/RConn1 -- Current Measurement/LConn1
  -/RConn1 -- Current Measurement/RConn1

== system parallel_modules_2_parasitic/Module 1/Subsystem9 ==
  Current Measurement : powerlib/Measurements/Current Measurement  PhasorSimulation=off  OutputType=Complex  PSBequivalent=0
  Scope : Scope
  + : PMIOPort  Side=Right
  - : PMIOPort  Port=2  Side=Left
  wires:
  Current Measurement/1 -> Scope/1
  connections:
  +/RConn1 -- Current Measurement/LConn1
  -/RConn1 -- Current Measurement/RConn1

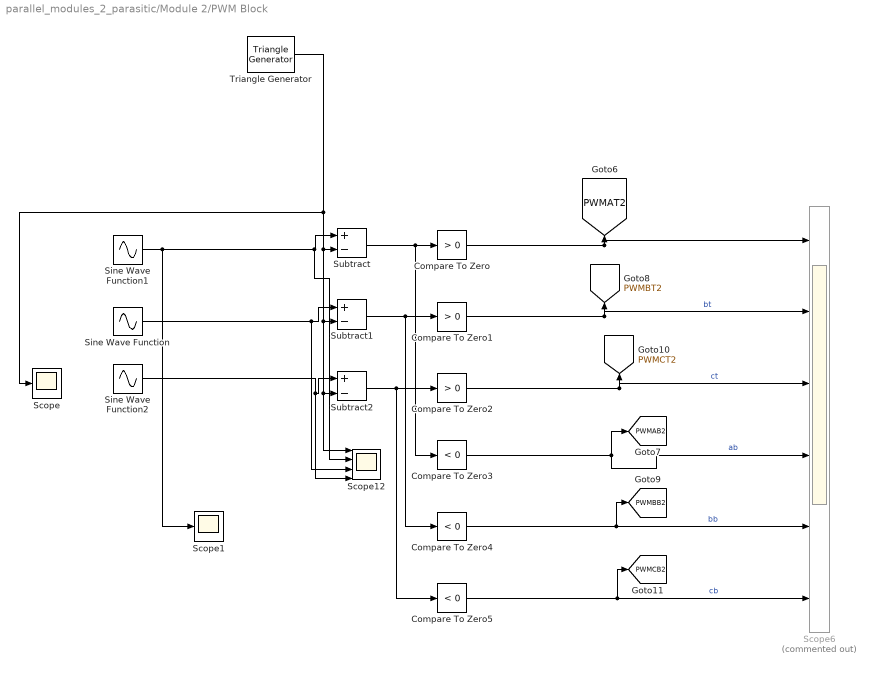
== system parallel_modules_2_parasitic/Module 2/PWM Block ==
  Compare To Zero : simulink/Logic and Bit Operations/Compare To Zero  relop=>  OutDataTypeStr=boolean
  Compare To Zero1 : simulink/Logic and Bit Operations/Compare To Zero  relop=>  OutDataTypeStr=boolean
  Compare To Zero2 : simulink/Logic and Bit Operations/Compare To Zero  relop=>  OutDataTypeStr=boolean
  Compare To Zero3 : simulink/Logic and Bit Operations/Compare To Zero  relop=<  OutDataTypeStr=boolean
  Compare To Zero4 : simulink/Logic and Bit Operations/Compare To Zero  relop=<  OutDataTypeStr=boolean
  Compare To Zero5 : simulink/Logic and Bit Operations/Compare To Zero  relop=<  OutDataTypeStr=boolean
  Scope : Scope
  Scope1 : Scope
  Scope12 : Scope  NumInputPorts=4
  Scope6 : Scope  Commented=on  NumInputPorts=6
  Sine Wave Function : Sin  Amplitude=ModulationIndex2  Frequency=ffund*2*pi  Phase=-2*pi/3  SampleTime=0
  Sine Wave Function1 : Sin  Amplitude=ModulationIndex2  Frequency=ffund*2*pi  SampleTime=0
  Sine Wave Function2 : Sin  Amplitude=ModulationIndex2  Frequency=ffund*2*pi  Phase=2*pi/3  SampleTime=0
  Subtract : Sum  Inputs=+-
  Subtract1 : Sum  Inputs=+-
  Subtract2 : Sum  Inputs=+-
  Triangle Generator : powerlib_meascontrol/Pulse & Signal Generators/Triangle Generator  Freq=fsw  Phase=Module2Phase  Ts=SampleTime
  tag scope: PWMAB2=global, PWMAT2=global, PWMBB2=global, PWMBT2=global, PWMCB2=global, PWMCT2=global
  wires:
  Compare To Zero2/1 -> [PWMCT2], Scope6/3  "ct"
  Sine Wave Function/1 -> Subtract1/1, Scope12/3
  Subtract2/1 -> Compare To Zero5/1, Compare To Zero2/1
  Sine Wave Function1/1 -> Scope1/1, Scope12/2, Subtract/1
  Subtract1/1 -> Compare To Zero4/1, Compare To Zero1/1
  Triangle Generator/1 -> Scope/1, Scope12/1, Subtract2/2, Subtract1/2, Subtract/2
  Compare To Zero/1 -> Scope6/1, [PWMAT2]
  Subtract/1 -> Compare To Zero3/1, Compare To Zero/1
  Compare To Zero1/1 -> [PWMBT2], Scope6/2  "bt"
  Compare To Zero5/1 -> [PWMCB2], Scope6/6  "cb"
  Compare To Zero4/1 -> [PWMBB2], Scope6/5  "bb"
  Sine Wave Function2/1 -> Scope12/4, Subtract2/1
  Compare To Zero3/1 -> [PWMAB2], Scope6/4  "ab"

== system parallel_modules_2_parasitic/Module 2/Subsystem ==
  Scope : Scope
  Voltage Measurement : powerlib/Measurements/Voltage Measurement  PhasorSimulation=off  OutputType=Complex  PSBequivalent=0
  + : PMIOPort  Side=Left
  - : PMIOPort  Port=2  Side=Left
  wires:
  Voltage Measurement/1 -> Scope/1
  connections:
  Voltage Measurement/LConn1 -- +/RConn1
  Voltage Measurement/LConn2 -- -/RConn1

== system parallel_modules_2_parasitic/Module 2/Subsystem1 ==
  Scope : Scope
  Voltage Measurement : powerlib/Measurements/Voltage Measurement  PhasorSimulation=off  OutputType=Complex  PSBequivalent=0
  + : PMIOPort  Side=Left
  - : PMIOPort  Port=2  Side=Left
  wires:
  Voltage Measurement/1 -> Scope/1
  connections:
  Voltage Measurement/LConn1 -- +/RConn1
  Voltage Measurement/LConn2 -- -/RConn1

== system parallel_modules_2_parasitic/Module 2/Subsystem10 ==
  Current Measurement : powerlib/Measurements/Current Measurement  PhasorSimulation=off  OutputType=Complex  PSBequivalent=0
  Scope : Scope
  + : PMIOPort  Side=Right
  - : PMIOPort  Port=2  Side=Left
  wires:
  Current Measurement/1 -> Scope/1
  connections:
  +/RConn1 -- Current Measurement/LConn1
  -/RConn1 -- Current Measurement/RConn1

== system parallel_modules_2_parasitic/Module 2/Subsystem11 ==
  Current Measurement : powerlib/Measurements/Current Measurement  PhasorSimulation=off  OutputType=Complex  PSBequivalent=0
  Scope : Scope
  + : PMIOPort  Side=Right
  - : PMIOPort  Port=2  Side=Left
  wires:
  Current Measurement/1 -> Scope/1
  connections:
  +/RConn1 -- Current Measurement/LConn1
  -/RConn1 -- Current Measurement/RConn1

== system parallel_modules_2_parasitic/Module 2/Subsystem12 ==
  Current Measurement : powerlib/Measurements/Current Measurement  PhasorSimulation=off  OutputType=Complex  PSBequivalent=0
  Scope : Scope
  + : PMIOPort  Side=Right
  - : PMIOPort  Port=2  Side=Left
  wires:
  Current Measurement/1 -> Scope/1
  connections:
  +/RConn1 -- Current Measurement/LConn1
  -/RConn1 -- Current Measurement/RConn1

== system parallel_modules_2_parasitic/Module 2/Subsystem13 ==
  Current Measurement : powerlib/Measurements/Current Measurement  PhasorSimulation=off  OutputType=Complex  PSBequivalent=0
  Scope : Scope
  + : PMIOPort  Side=Right
  - : PMIOPort  Port=2  Side=Left
  wires:
  Current Measurement/1 -> Scope/1
  connections:
  +/RConn1 -- Current Measurement/LConn1
  -/RConn1 -- Current Measurement/RConn1

== system parallel_modules_2_parasitic/Module 2/Subsystem2 ==
  Scope : Scope
  Voltage Measurement : powerlib/Measurements/Voltage Measurement  PhasorSimulation=off  OutputType=Complex  PSBequivalent=0
  + : PMIOPort  Side=Left
  - : PMIOPort  Port=2  Side=Left
  wires:
  Voltage Measurement/1 -> Scope/1
  connections:
  Voltage Measurement/LConn1 -- +/RConn1
  Voltage Measurement/LConn2 -- -/RConn1

== system parallel_modules_2_parasitic/Module 2/Subsystem3 ==
  Current Measurement : powerlib/Measurements/Current Measurement  PhasorSimulation=off  OutputType=Complex  PSBequivalent=0
  Scope : Scope
  + : PMIOPort  Side=Right
  - : PMIOPort  Port=2  Side=Left
  wires:
  Current Measurement/1 -> Scope/1
  connections:
  +/RConn1 -- Current Measurement/LConn1
  -/RConn1 -- Current Measurement/RConn1

== system parallel_modules_2_parasitic/Module 2/Subsystem4 ==
  Current Measurement : powerlib/Measurements/Current Measurement  PhasorSimulation=off  OutputType=Complex  PSBequivalent=0
  Scope : Scope
  + : PMIOPort  Side=Right
  - : PMIOPort  Port=2  Side=Left
  wires:
  Current Measurement/1 -> Scope/1
  connections:
  +/RConn1 -- Current Measurement/LConn1
  -/RConn1 -- Current Measurement/RConn1

== system parallel_modules_2_parasitic/Module 2/Subsystem5 ==
  Current Measurement : powerlib/Measurements/Current Measurement  PhasorSimulation=off  OutputType=Complex  PSBequivalent=0
  Scope : Scope
  + : PMIOPort  Side=Right
  - : PMIOPort  Port=2  Side=Left
  wires:
  Current Measurement/1 -> Scope/1
  connections:
  +/RConn1 -- Current Measurement/LConn1
  -/RConn1 -- Current Measurement/RConn1

== system parallel_modules_2_parasitic/Module 2/Subsystem8 ==
  Current Measurement : powerlib/Measurements/Current Measurement  PhasorSimulation=off  OutputType=Complex  PSBequivalent=0
  Scope : Scope
  + : PMIOPort  Side=Right
  - : PMIOPort  Port=2  Side=Left
  wires:
  Current Measurement/1 -> Scope/1
  connections:
  +/RConn1 -- Current Measurement/LConn1
  -/RConn1 -- Current Measurement/RConn1

== system parallel_modules_2_parasitic/Module 2/Subsystem9 ==
  Current Measurement : powerlib/Measurements/Current Measurement  PhasorSimulation=off  OutputType=Complex  PSBequivalent=0
  Scope : Scope
  + : PMIOPort  Side=Right
  - : PMIOPort  Port=2  Side=Left
  wires:
  Current Measurement/1 -> Scope/1
  connections:
  +/RConn1 -- Current Measurement/LConn1
  -/RConn1 -- Current Measurement/RConn1
